simulink model "mpc_setup_2021b"  (R2021b)
settings: Solver=VariableStepAuto  StartTime=0.0  StopTime=40  RelTol=1e-3
undefined symbols (not defined in the file or in its folder): MPCparams
libraries: simulink x1
settings Model: Creator=liaml  LastModifiedBy=liamligthart
settings DebuggingCC: UnconnectedInputMsg=none  UnconnectedOutputMsg=none  UnconnectedLineMsg=none
settings ModelReferenceCC: EnableRefExpFcnMdlSchedulingChecks=off
settings RTWCC: DLArmComputeVersion=20.02.1

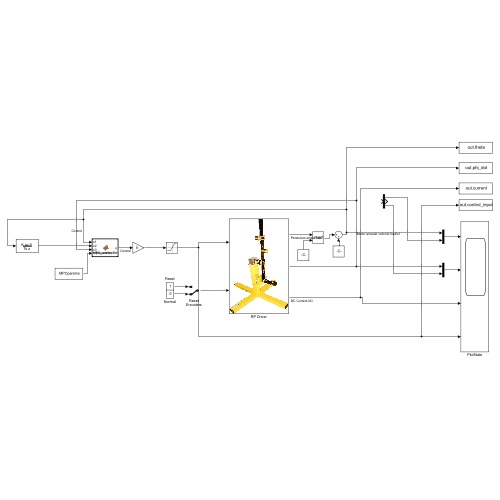
[thumbnail: Simulink's stored preview of the top-level diagram]
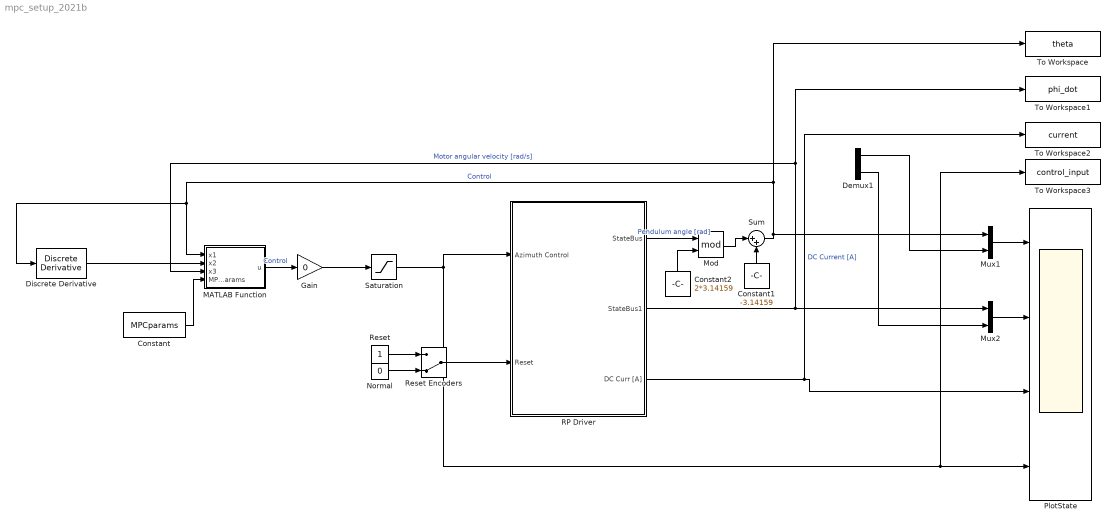
== system mpc_setup_2021b ==
  Constant : Constant  Value=MPCparams  OutDataTypeStr=Bus: MPCparams_bus
  Constant1 : Constant  Value=-3.14159
  Constant2 : Constant  Value=2*3.14159
  Demux1 : Demux  Outputs=3
  Discrete Derivative : simulink/Discrete/Discrete Derivative  gainval=1.0  ICPrevScaledInput=0.0  OutMin=[]  OutMax=[]  OutDataType=fixdt(1, 16)  OutScaling=2^-10  DoSatur=off
  Gain : Gain  Gain=0
  MATLAB Function : MATLAB Function  TreatAsAtomicUnit=on
  Mod : Math  Operator=mod  SaturateOnIntegerOverflow=on
  Mux1 : Mux  Inputs=2
  Mux2 : Mux  Inputs=2
  Normal : Constant  Value=0
  PlotState : Scope  NumInputPorts=4
  RP Driver : Subsystem
      mask Display: image(imread('rwp.JPG'))
  Reset : Constant
  Reset Encoders : ManualSwitch  CurrentSetting=0
  Saturation : Saturate  UpperLimit=1  LowerLimit=-1
  Sum : Sum  Inputs=|++
  To Workspace : ToWorkspace  VariableName=theta  SaveFormat=Timeseries  SampleTime=-1
  To Workspace1 : ToWorkspace  VariableName=phi_dot  SaveFormat=Timeseries  SampleTime=-1
  To Workspace2 : ToWorkspace  VariableName=current  SaveFormat=Timeseries  SampleTime=-1
  To Workspace3 : ToWorkspace  VariableName=control_input  SaveFormat=Timeseries  SampleTime=-1
  wires:
  MATLAB Function/1(u) -> Gain/1  "Control"
  Constant/1 -> MATLAB Function/4(MPCparams)
  RP Driver/2(StateBus1) -> To Workspace1/1, MATLAB Function/3(x3), Mux2/1  "Motor angular velocity [rad/s]"
  Mux1/1 -> PlotState/1
  Mux2/1 -> PlotState/2
  Demux1/3 -> Mux2/2
  RP Driver/3(DC Curr [A]) -> To Workspace2/1, PlotState/3  "DC Current [A]"
  Saturation/1 -> RP Driver/1(Azimuth Control), To Workspace3/1, PlotState/4
  Constant1/1 -> Sum/2
  RP Driver/1(StateBus) -> Mod/1  "Pendulum angle [rad]"
  Mod/1 -> Sum/1
  Constant2/1 -> Mod/2
  Reset Encoders/1 -> RP Driver/2(Reset)
  Normal/1 -> Reset Encoders/2
  Reset/1 -> Reset Encoders/1
  Demux1/1 -> Mux1/2
  Gain/1 -> Saturation/1
  Sum/1 -> Discrete Derivative/1, MATLAB Function/1(x1), To Workspace/1, Mux1/1  "Control"
  Discrete Derivative/1 -> MATLAB Function/2(x2)

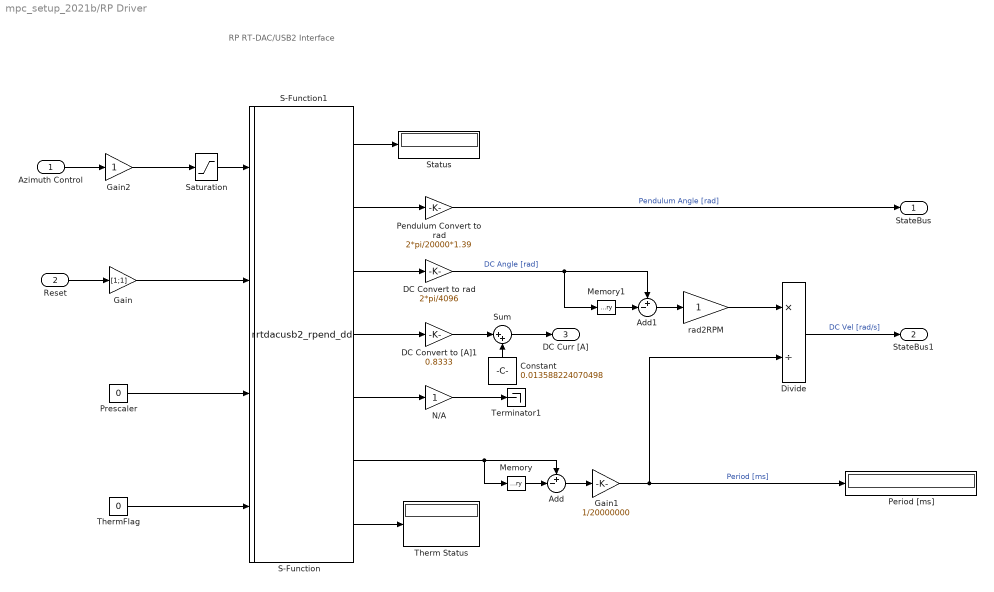
== system mpc_setup_2021b/RP Driver ==
  note: RP RT-DAC/USB2
      | Interface
  Azimuth Control : Inport
  Reset : Inport  Port=2
  Add : Sum  Inputs=+-|
  Add1 : Sum  Inputs=+-|
  Constant : Constant  Value=0.013588224070498
  DC Convert to [A]1 : Gain  Gain=0.8333  SaturateOnIntegerOverflow=on  OutDataTypeStr=Inherit: Same as input  ParamDataTypeStr=Inherit: Same as input
  DC Convert to rad : Gain  Gain=2*pi/4096  SaturateOnIntegerOverflow=on  OutDataTypeStr=Inherit: Same as input  ParamDataTypeStr=Inherit: Same as input
  Divide : Product  Inputs=*/
  Gain : Gain  Gain=[1;1]
  Gain1 : Gain  Gain=1/20000000
  Gain2 : Gain
  Memory : Memory
  Memory1 : Memory
  N/A : Gain  SaturateOnIntegerOverflow=on  OutDataTypeStr=Inherit: Same as input  ParamDataTypeStr=Inherit: Same as input
  Pendulum Convert to rad : Gain  Gain=2*pi/20000*1.39  SaturateOnIntegerOverflow=on  OutDataTypeStr=Inherit: Same as input  ParamDataTypeStr=Inherit: Same as input
  Period [ms] : Display
  Prescaler : Constant  Value=0
  S-Function : S-Function  Priority=1  FunctionName=rtdacusb2_rpend_dd  Parameters=1, h  SFunctionDeploymentMode=off  EnableBusSupport=off
  S-Function1 : S-Function  FunctionName=rtdacusb2_rpend_dd  Parameters=1, h  SFunctionDeploymentMode=off  EnableBusSupport=off
  Saturation : Saturate  UpperLimit=1  LowerLimit=-1
  Status : Display
  Sum : Sum  Inputs=|++
  Terminator1 : Terminator
  Therm Status : Display
  ThermFlag : Constant  Value=0
  rad2RPM : Gain  SaturateOnIntegerOverflow=on  OutDataTypeStr=Inherit: Same as input  ParamDataTypeStr=Inherit: Same as input
  StateBus : Outport  VectorParamsAs1DForOutWhenUnconnected=off
  StateBus1 : Outport  Port=2  VectorParamsAs1DForOutWhenUnconnected=off
  DC Curr [A] : Outport  Port=3  VectorParamsAs1DForOutWhenUnconnected=off
  wires:
  S-Function/7 -> Therm Status/1
  S-Function/5 -> N/A/1
  S-Function/4 -> DC Convert to [A]1/1
  ThermFlag/1 -> S-Function/4
  Prescaler/1 -> S-Function/3
  Gain/1 -> S-Function/2
  Divide/1 -> StateBus1/1  "DC Vel [rad/s]"
  rad2RPM/1 -> Divide/1
  Add1/1 -> rad2RPM/1
  Memory1/1 -> Add1/2
  N/A/1 -> Terminator1/1
  S-Function/6 -> Add/1, Memory/1
  Gain2/1 -> Saturation/1
  Gain1/1 -> Period [ms]/1, Divide/2  "Period [ms]"
  Add/1 -> Gain1/1
  Memory/1 -> Add/2
  DC Convert to rad/1 -> Add1/1, Memory1/1  "DC Angle [rad]"
  S-Function/3 -> DC Convert to rad/1
  Pendulum Convert to rad/1 -> StateBus/1  "Pendulum Angle [rad]"
  S-Function/2 -> Pendulum Convert to rad/1
  S-Function/1 -> Status/1
  Saturation/1 -> S-Function/1
  Reset/1 -> Gain/1
  Azimuth Control/1 -> Gain2/1
  DC Convert to [A]1/1 -> Sum/1
  Sum/1 -> DC Curr [A]/1
  Constant/1 -> Sum/2

== matlab function mpc_setup_2021b/MATLAB Function ==
  data: x1 input; x2 input; x3 input; u output; MPCparams input
function u = mpc_controller(x1, x2, x3, MPCparams)
    % Inputs:
    % x:            observer state at current time [nx x 1]
    % MPCparams:    struct with all offline MPC calculations
    %
    % Outputs:
    % u:            optimal input at current time [1 x 1]
    
    % Initialize u
    u = zeros(1,1);
    
    x3(isnan(x3)) = 0;
    x3(isinf(x3)) = 0;

    x = [x1; x2; x3];
    disp(x);
    disp("next iteration");

    % Compute linear part of cost function (dependent on x0)
    f_i = MPCparams.CostMatrices.f * x;

    % Compute bound vector on u (dependent on x0)
    b_i = [MPCparams.Bounds.bx - MPCparams.Bounds.Ax * MPCparams.PredMatrices.T * x; MPCparams.Bounds.bu];
    
    % Do the optimization
    %coder.extrinsic('quadprog');
    [u_opt, ~, exitflag, ~] = quadprog(MPCparams.CostMatrices.H, f_i, MPCparams.Bounds.A, b_i, [], [], [], [], zeros(size(f_i)), optimoptions('quadprog', Display='off', Algorithm='active-set'));

    if exitflag ~= 1
        disp("WARNING: exitflag = " + exitflag);
    end
    u = u_opt(1);

end
